simulink model "PoseExecutor"  (R2019b)
settings: Solver=FixedStepDiscrete  StartTime=0.0  StopTime=datatime_end  FixedStep=.05  RelTol=1e-3
libraries: posemodel x1

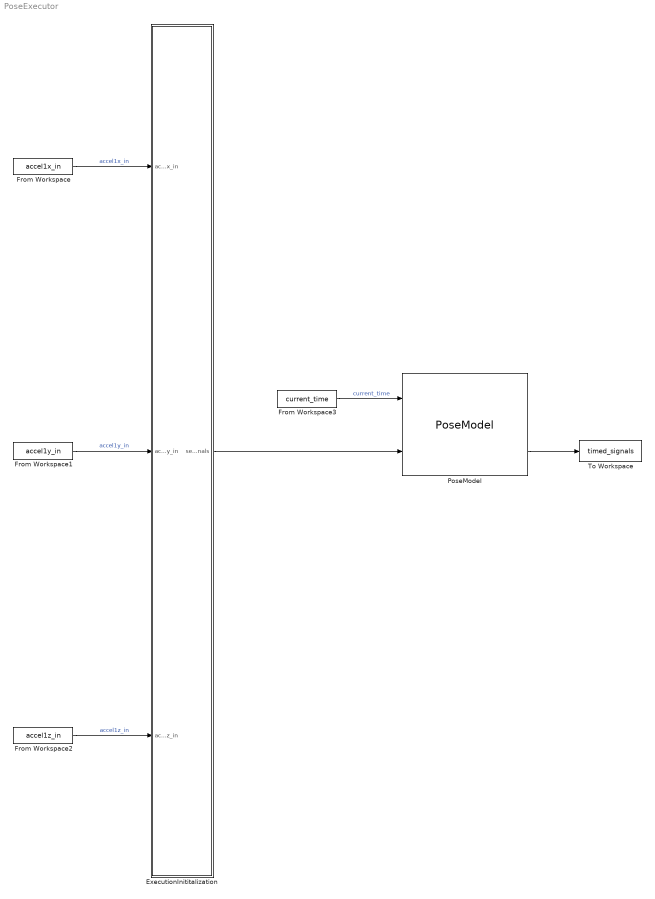
== system PoseExecutor ==
  ExecutionInititalization : Subsystem  AncestorBlock=posemodel/ExecutionInititalization
  From Workspace : FromWorkspace  VariableName=accel1x_in  SampleTime=0
  From Workspace1 : FromWorkspace  VariableName=accel1y_in  SampleTime=0
  From Workspace2 : FromWorkspace  VariableName=accel1z_in  SampleTime=0
  From Workspace3 : FromWorkspace  VariableName=current_time  SampleTime=0
  PoseModel : posemodel/PoseModel  SystemSampleTime=-1  Latency=0  AutoFrameSizeCalculation=off
  To Workspace : ToWorkspace  VariableName=timed_signals  SaveFormat=Timeseries  SampleTime=-1
  wires:
  From Workspace/1 -> ExecutionInititalization/1(accel1x_in)  "accel1x_in"
  From Workspace1/1 -> ExecutionInititalization/2(accel1y_in)  "accel1y_in"
  From Workspace2/1 -> ExecutionInititalization/3(accel1z_in)  "accel1z_in"
  ExecutionInititalization/1(sensor_signals) -> PoseModel/2
  PoseModel/2 -> To Workspace/1
  From Workspace3/1 -> PoseModel/1  "current_time"

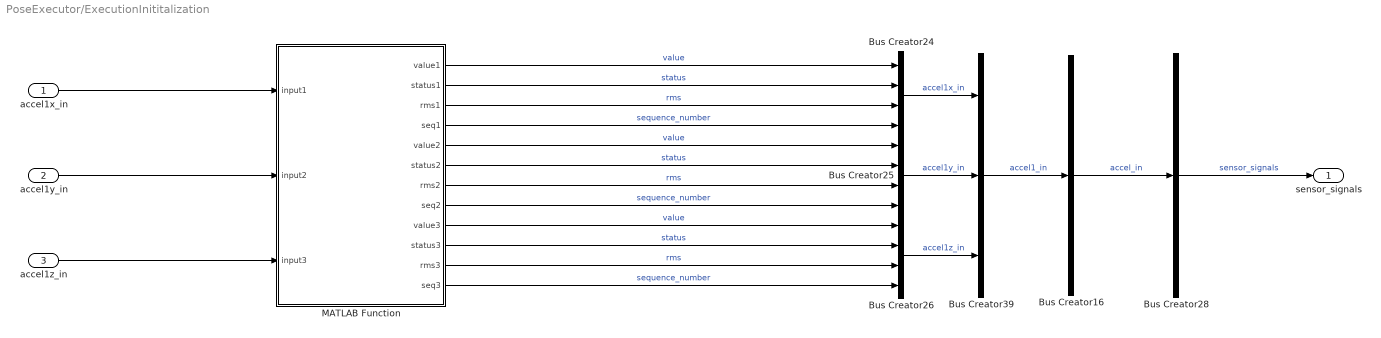
== system PoseExecutor/ExecutionInititalization ==
  accel1x_in : Inport
  accel1y_in : Inport  Port=2
  accel1z_in : Inport  Port=3
  Bus Creator16 : BusCreator  Inputs=1
  Bus Creator24 : BusCreator  Inputs=4  OutDataTypeStr=Bus: InputSignalObject
  Bus Creator25 : BusCreator  Inputs=4  OutDataTypeStr=Bus: InputSignalObject
  Bus Creator26 : BusCreator  Inputs=4  OutDataTypeStr=Bus: InputSignalObject
  Bus Creator28 : BusCreator  Inputs=1
  Bus Creator39 : BusCreator  Inputs=3
  MATLAB Function : MATLAB Function  TreatAsAtomicUnit=on
  sensor_signals : Outport
  wires:
  MATLAB Function/10(status3) -> Bus Creator26/2  "status"
  MATLAB Function/1(value1) -> Bus Creator24/1  "value"
  accel1y_in/1 -> MATLAB Function/2(input2)
  Bus Creator26/1 -> Bus Creator39/3  "accel1z_in"
  MATLAB Function/8(seq2) -> Bus Creator25/4  "sequence_number"
  MATLAB Function/7(rms2) -> Bus Creator25/3  "rms"
  MATLAB Function/9(value3) -> Bus Creator26/1  "value"
  Bus Creator25/1 -> Bus Creator39/2  "accel1y_in"
  Bus Creator16/1 -> Bus Creator28/1  "accel_in"
  Bus Creator24/1 -> Bus Creator39/1  "accel1x_in"
  accel1z_in/1 -> MATLAB Function/3(input3)
  MATLAB Function/6(status2) -> Bus Creator25/2  "status"
  accel1x_in/1 -> MATLAB Function/1(input1)
  Bus Creator28/1 -> sensor_signals/1  "sensor_signals"
  Bus Creator39/1 -> Bus Creator16/1  "accel1_in"
  MATLAB Function/12(seq3) -> Bus Creator26/4  "sequence_number"
  MATLAB Function/11(rms3) -> Bus Creator26/3  "rms"
  MATLAB Function/4(seq1) -> Bus Creator24/4  "sequence_number"
  MATLAB Function/2(status1) -> Bus Creator24/2  "status"
  MATLAB Function/5(value2) -> Bus Creator25/1  "value"
  MATLAB Function/3(rms1) -> Bus Creator24/3  "rms"

== matlab function PoseExecutor/ExecutionInititalization/MATLAB Function ==
function [value1,status1,rms1,seq1, ... 
            value2,status2,rms2,seq2, ... 
            value3,status3,rms3,seq3] ...
              = inputdata_tobus_x3( ...
                input1,input2,input3)
VALUE_INDEX = 1;
STATUS_INDEX = 2;
RMS_INDEX = 3;
SEQUENCENUMBER_INDEX = 4;

value1 = input1(VALUE_INDEX);
status1 = uint8(input1(STATUS_INDEX));
rms1 = input1(RMS_INDEX);
seq1 = uint32(input1(SEQUENCENUMBER_INDEX));

value2 = input2(VALUE_INDEX);
status2 = uint8(input2(STATUS_INDEX));
rms2 = input2(RMS_INDEX);
seq2 = uint32(input2(SEQUENCENUMBER_INDEX));

value3 = input3(VALUE_INDEX);
status3 = uint8(input3(STATUS_INDEX));
rms3 = input3(RMS_INDEX);
seq3 = uint32(input3(SEQUENCENUMBER_INDEX));
end
